simulink model "half_car_model_active_suspension"  (R2023b)
settings: Solver=VariableStepAuto  StartTime=0.0  StopTime=20.0  RelTol=1e-3
values from neighbouring files (symbols this model uses):
  x0 = [  2 ... (first row only)    [half_car_active_suspensions.m]
settings Model: Creator=alex2  LastModifiedBy=alex2

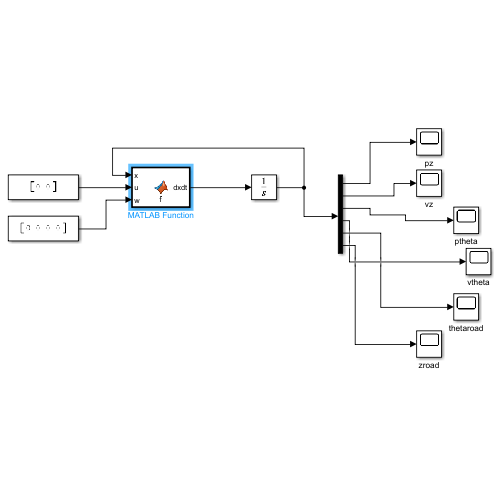
[thumbnail: Simulink's stored preview of the top-level diagram]
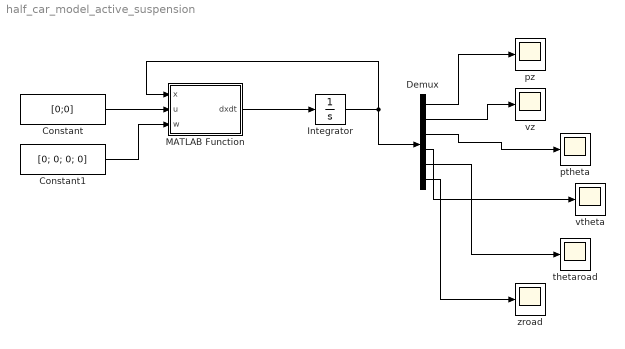
== system half_car_model_active_suspension ==
  Constant : Constant  Value=[0;0]
  Constant1 : Constant  Value=[0; 0; 0; 0]
  Demux : Demux  Outputs=6
  Integrator : Integrator  InitialCondition=x0
  MATLAB Function : MATLAB Function  TreatAsAtomicUnit=on
  ptheta : Scope
  pz : Scope
  thetaroad : Scope
  vtheta : Scope
  vz : Scope
  zroad : Scope
  wires:
  MATLAB Function/1(dxdt) -> Integrator/1
  Integrator/1 -> Demux/1, MATLAB Function/1(x)
  Constant/1 -> MATLAB Function/2(u)
  Constant1/1 -> MATLAB Function/3(w)
  Demux/1 -> pz/1
  Demux/2 -> vz/1
  Demux/3 -> ptheta/1
  Demux/4 -> vtheta/1
  Demux/5 -> thetaroad/1
  Demux/6 -> zroad/1

== matlab function half_car_model_active_suspension/MATLAB Function ==
  data: x input; u input; dxdt output; w input
function dxdt = f(x,u,w)
%% parameters
m = 400;      % [kg] mass
k = 170000;    % [N/m] spring stiffness
beta = 15000;   % [N/(m/s)] damper coeff.
ell0 = 0.3;   % [m] 0-load lenght
g = 9.81;   % [m/s^2] gravity acceleration
df = 2;     % [m] distance between center of mass and front
dr = 1.5;     % [m] distance between center of mass and rear
J = 400;      % [kg*m^2] Moment of intertia 
%% state
pz = x(1);        % [m] heigth of the center of mass of the car 
vz = x(2);        % [m/s] speed of the center of mass of the car 
ptheta = x(3);    % [Rad] pitch angle of the car 
vtheta = x(4);    % [Rad/s] angular speed of the car 
thetaroad = x(5); % [Rad]Road slope
zroad = x(6);     %[m]Road height 

%% disturbance
zgsecond = w(1);
alphag = w(2);
fwfront = w(3);
fwrear = w(4);

%todo: Vedere se servono due disturbi 

%% state evolution

s1 = pz+df*(sin(ptheta)-sin(thetaroad)); % height of front suspension
s3 = pz-dr*(sin(ptheta)-sin(thetaroad)); % height of rear suspension

s2 = vz+df*(vtheta*cos(ptheta)-zroad*cos(thetaroad)); % height speed of front suspension
s4 = vz-dr*(vtheta*cos(ptheta)-zroad*cos(thetaroad)); % height speed of rear suspension

lf = s1 + ell0;
lr = s3 + ell0;

f2 = -g + (((-k*(s1-ell0)-beta*s2)+(-k*(s3-ell0)-beta*s4))+u(1))/m; %  con
%ell0
f4 = (df*(-k*(s1-ell0)-beta*s2)-dr*(-k*(s3-ell0)-beta*s4)+u(2)+fwfront*lf+fwrear*lr)/J; %

%f2 = -g + (((-k*(s1)-beta*s2)+(-k*(s3)-beta*s4))+u(1))/m; % 
%f4 = (df*(-k*(s1)-beta*s2)-dr*(-k*(s3)-beta*s4)+u(2)+fwfront*lf+fwrear*lr)/J; %

dxdt = [vz;
        f2-zgsecond; 
        x(4);
        f4;
        x(6);
        alphag];
        




end
